simulink model "polar_nrz"  (Simulink 8.7)
settings: Solver=ode5  SolverMode=SingleTasking  StartTime=0.0  StopTime=1  FixedStep=1/fs  RelTol=1e-3  AbsTol=1e-6
PreLoadFcn:
  | R=1000; fs=10*R;
undefined symbols (not defined in the file or in its folder): bessel_den, bessel_num
libraries: commnoisgen2 x1, commrandsrc2 x1
settings Model: Creator=amoura  LastModifiedBy=Artur Moura
settings DataIOCC: LimitDataPoints=off  SignalLoggingSaveFormat=ModelDataLogs  SignalLoggingName=sigsOut
settings OptimizationCC: BooleanDataType=off  ExpressionDepthLimit=2147483647  InitFltsAndDblsToZero=on
settings DebuggingCC: SaveWithParameterizedLinksMsg=none  SignalResolutionControl=TryResolveAllWithWarning  MultiTaskDSMMsg=warning  MultiTaskCondExecSysMsg=none  FcnCallInpInsideContextMsg=UseLocalSettings  StateNameClashWarn=warning
settings HardwareCC: TargetUnknown=on
settings RTWCC: TemplateMakefile=grt_unix.tmf
settings GRTTargetCC: TargetFcnLib=ansi_tfl_tmw.mat  ModelReferenceCompliant=off  CombineOutputUpdateFcns=off  MatFileLogging=off  GRTInterface=on

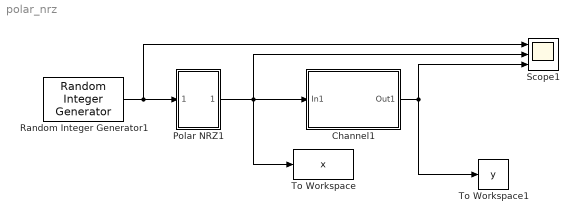
== system polar_nrz ==
  Channel1 : Subsystem  mask(Communications channel){gain=1, bw=4000, noise_pwr=.01, noise_seed=123}
      mask prompts: bw "Bandwidth (Hz):"; noise_pwr "Noise power:"; noise_seed "Noise seed:"
      mask init:
      | [bessel_num, bessel_den]=besself(8,2*pi*bw);
      | if noise_pwr==0 , noise_var=1e-20; else noise_var=noise_pwr; end
      mask Display: disp('Communications\nchannel')
  Polar NRZ1 : Subsystem  mask(Polar NRZ){}
      mask help:
      | This block encodes a unipolar NRZ signal into the polar NRZ line code
      |
      | The output values are +1 for a nonzero input and -1 for a zero one.
      mask Display: disp('Polar\nNRZ')
  Random Integer Generator1 : commrandsrc2/Random Integer Generator  mul=2  seed=37  Ts=1/R  frameBased=off  sampPerFrame=1  orient=on  outDataType=double
  Scope1 : Scope  NumInputPorts=3
  To Workspace : ToWorkspace  VariableName=x  SampleTime=1/fs
  To Workspace1 : ToWorkspace  VariableName=y  SampleTime=1/fs
  wires:
  Channel1/1(Out1) -> To Workspace1/1, Scope1/3
  Random Integer Generator1/1 -> Scope1/1, Polar NRZ1/1(In1)
  Polar NRZ1/1(Out1) -> Channel1/1(In1), To Workspace/1, Scope1/2

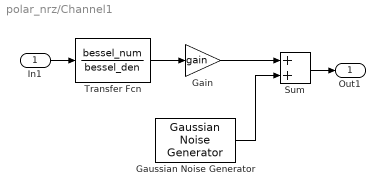
== system polar_nrz/Channel1 ==
  In1 : Inport
  Gain : Gain  Gain=gain  SaturateOnIntegerOverflow=on  OutDataTypeStr=Inherit: Same as input  ParamDataTypeStr=Inherit: Same as input
  Gaussian Noise Generator : commnoisgen2/Gaussian Noise Generator  m=0  d=noise_pwr  s=noise_seed  Ts=1/fs  frameBased=off  sampPerFrame=1  orient=on  outDataType=double
  Sum : Sum  SaturateOnIntegerOverflow=on  InputSameDT=on  OutDataTypeStr=Inherit: Same as first input
  Transfer Fcn : TransferFcn  Numerator=bessel_num  Denominator=bessel_den
  Out1 : Outport
  wires:
  Sum/1 -> Out1/1
  In1/1 -> Transfer Fcn/1
  Transfer Fcn/1 -> Gain/1
  Gain/1 -> Sum/1
  Gaussian Noise Generator/1 -> Sum/2

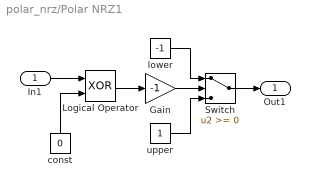
== system polar_nrz/Polar NRZ1 ==
  In1 : Inport
  Gain : Gain  Gain=-1  SaturateOnIntegerOverflow=on  OutDataTypeStr=Inherit: Same as input  ParamDataTypeStr=Inherit: Same as input
  Logical Operator : Logic  Operator=XOR
  Switch : Switch  SaturateOnIntegerOverflow=on  InputSameDT=on
  const : Constant  Value=0
  lower : Constant  Value=-1
  upper : Constant
  Out1 : Outport
  wires:
  In1/1 -> Logical Operator/1
  lower/1 -> Switch/1
  upper/1 -> Switch/3
  Gain/1 -> Switch/2
  Switch/1 -> Out1/1
  Logical Operator/1 -> Gain/1
  const/1 -> Logical Operator/2
